simulink model "pendule_inverse"  (Simulink 7.5)
settings: Solver=ode45  StartTime=0.0  StopTime=inf  RelTol=1e-3
libraries: vrlib x1
settings Model: Creator=Administrateur  LastModifiedBy=vidub
settings OptimizationCC: InitFltsAndDblsToZero=on
settings DebuggingCC: StrictBusMsg=Warning

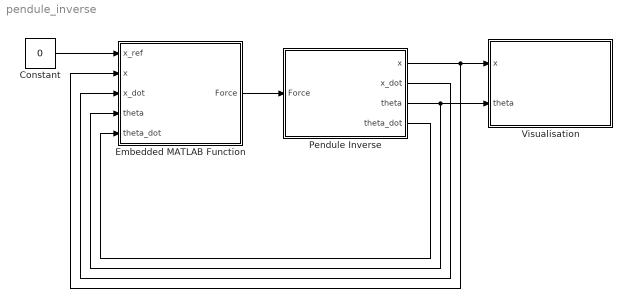
== system pendule_inverse ==
  Constant : Constant  Value=0  OutDataType=fixdt(1, 16)  OutScaling=2^0
  Embedded MATLAB Function : Stateflow chart  TreatAsAtomicUnit=on
  Pendule Inverse : Subsystem
  Visualisation : Subsystem
  wires:
  Pendule Inverse/1(x) -> Visualisation/1(x), Embedded MATLAB Function/2(x)
  Pendule Inverse/3("theta ") -> Visualisation/2(theta), Embedded MATLAB Function/4(theta)
  Embedded MATLAB Function/1(Force) -> Pendule Inverse/1(Force)
  Constant/1 -> Embedded MATLAB Function/1(x_ref)
  Pendule Inverse/2("x_dot ") -> Embedded MATLAB Function/3(x_dot)
  Pendule Inverse/4("theta_dot ") -> Embedded MATLAB Function/5(theta_dot)

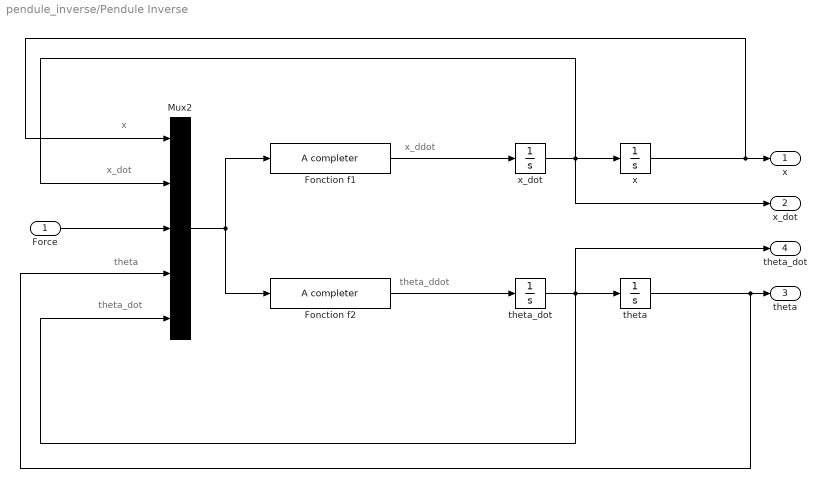
== system pendule_inverse/Pendule Inverse ==
  note: x
  note: x_dot
  note: theta
  note: theta_dot
  note: x_ddot
  note: theta_ddot
  Force : Inport
  " theta_dot" : Integrator
  " x_dot" : Integrator
  Fonction f1 : Fcn  Expr=A completer
  Fonction f2 : Fcn  Expr=A completer
  Mux2 : Mux  Inputs=5
  theta : Integrator  LimitOutput=on  UpperSaturationLimit=pi/2  LowerSaturationLimit=-pi/2
  "x " : Integrator  LimitOutput=on  UpperSaturationLimit=9.5  LowerSaturationLimit=-9.5
  x : Outport
  "x_dot " : Outport  Port=2
  "theta " : Outport  Port=3
  "theta_dot " : Outport  Port=4
  wires:
  Fonction f1/1 -> " x_dot"/1
  " x_dot"/1 -> "x "/1, Mux2/2, "x_dot "/1
  "x "/1 -> Mux2/1, x/1
  Mux2/1 -> Fonction f1/1, Fonction f2/1
  Fonction f2/1 -> " theta_dot"/1
  " theta_dot"/1 -> theta/1, "theta_dot "/1, Mux2/5
  theta/1 -> "theta "/1, Mux2/4
  Force/1 -> Mux2/3

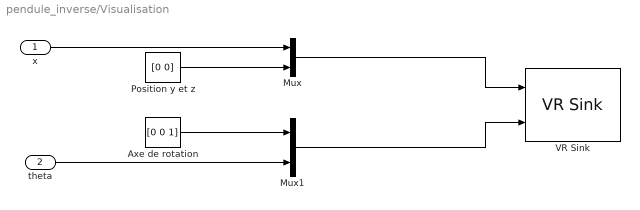
== system pendule_inverse/Visualisation ==
  x : Inport
  theta : Inport  Port=2
  Axe de rotation : Constant  Value=[0 0 1]  OutDataType=sfix(16)  OutScaling=2^0
  Mux : Mux  Inputs=2
  Mux1 : Mux  Inputs=2
  Position y et z : Constant  Value=[0 0]  OutDataType=sfix(16)  OutScaling=2^0
  VR Sink : vrlib/VR Sink  InstantiateOnLoad=on  SampleTime=0.1  ViewEnable=on  RemoteChange=off  RemoteView=on  FieldsWritten=Chariot.translation.3.1.1.double#Tige.rotation.4.1.1.double  WorldFileName=pendule_inverse.wrl  AutoView=off  VideoDimensions=[]
  wires:
  Mux/1 -> VR Sink/1
  Mux1/1 -> VR Sink/2
  x/1 -> Mux/1
  Axe de rotation/1 -> Mux1/1
  theta/1 -> Mux1/2
  Position y et z/1 -> Mux/2

== matlab function Embedded MATLAB Function ==
  data: x_ref input double; x input double; Force output double; x_dot input double; theta input double; theta_dot input double
function Force = fcn(x_ref,x,x_dot,theta,theta_dot)
% This block supports the Embedded MATLAB subset.
% See the help menu for details. 

Force = 0;
